simulink model "TargetTrackingRobotEnv"  (R2025a)
settings: Solver=VariableStepAuto  StartTime=0.0  StopTime=10.0  RelTol=1e-3
undefined symbols (not defined in the file): theta0, x0, y0
libraries: rllib x1
settings Model: Creator=ex  LastModifiedBy=ex

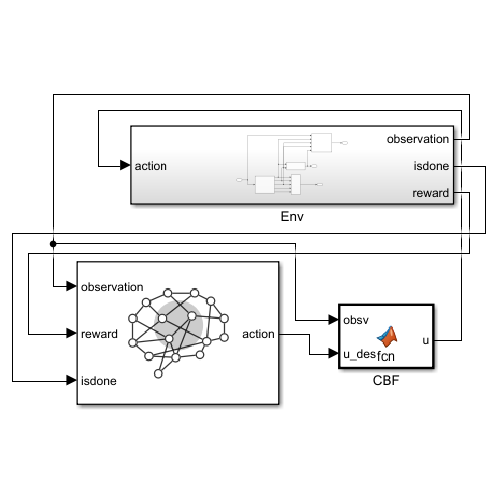
[thumbnail: Simulink's stored preview of the top-level diagram]
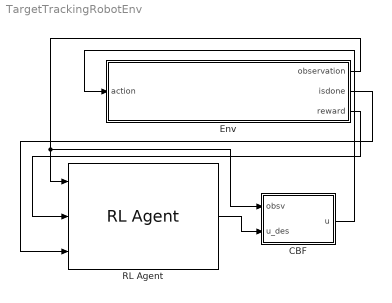
== system TargetTrackingRobotEnv ==
  CBF : MATLAB Function  TreatAsAtomicUnit=on
  Env : Subsystem
  RL Agent : rllib/RL Agent  Agent=agent  ExternalActionAsInput=off  ProvideLastAction=off  ProvideCumRwd=off  TreatAsDirectFeedthrough=on  UseStrictObservationDataTypes=off
  wires:
  Env/2(isdone) -> RL Agent/3
  Env/3(reward) -> RL Agent/2
  Env/1(observation) -> CBF/1(obsv), RL Agent/1
  RL Agent/1 -> CBF/2(u_des)
  CBF/1(u) -> Env/1(action)

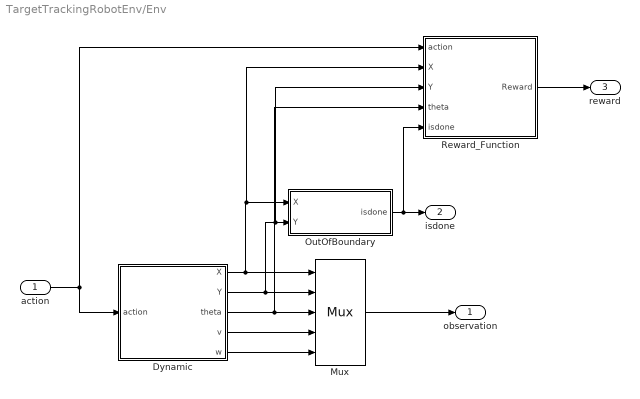
== system TargetTrackingRobotEnv/Env ==
  action : Inport
  Dynamic : Subsystem
  Mux : Mux  Inputs=5
  OutOfBoundary : Subsystem
  Reward_Function : Subsystem
  observation : Outport
  isdone : Outport  Port=2
  reward : Outport  Port=3
  wires:
  action/1 -> Reward_Function/1(action), Dynamic/1(action)
  Dynamic/1(X) -> Reward_Function/2(X), OutOfBoundary/1(X), Mux/1
  Dynamic/2(Y) -> Reward_Function/3(Y), OutOfBoundary/2(Y), Mux/2
  Dynamic/3(theta) -> Mux/3, Reward_Function/4(theta)
  Mux/1 -> observation/1
  OutOfBoundary/1(isdone) -> Reward_Function/5(isdone), isdone/1
  Reward_Function/1(Reward) -> reward/1
  Dynamic/4(v) -> Mux/4
  Dynamic/5(w) -> Mux/5

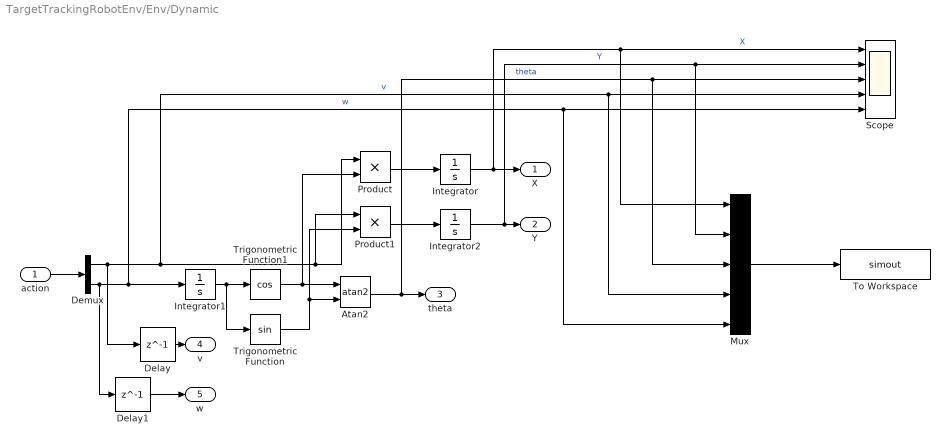
== system TargetTrackingRobotEnv/Env/Dynamic ==
  action : Inport
  Atan2 : Trigonometry  Operator=atan2
  Delay : Delay  DelayLength=1  InitialCondition=0
  Delay1 : Delay  DelayLength=1  InitialCondition=0
  Demux : Demux  Outputs=2
  Integrator : Integrator  InitialCondition=x0
  Integrator1 : Integrator  InitialCondition=theta0
  Integrator2 : Integrator  InitialCondition=y0
  Mux : Mux  Inputs=5
  Product : Product
  Product1 : Product
  Scope : Scope  NumInputPorts=5
      settings: ActiveDisplayYMinimum=-43.864327888983752  ActiveDisplayYMaximum=26.655261812730853
  To Workspace : ToWorkspace  VariableName=simout  SaveFormat=Structure With Time  SampleTime=-1
  Trigonometric Function : Trigonometry
  Trigonometric Function1 : Trigonometry  Operator=cos
  X : Outport
  Y : Outport  Port=2
  theta : Outport  Port=3
  v : Outport  Port=4
  w : Outport  Port=5
  wires:
  Trigonometric Function1/1 -> Product/2, Atan2/1
  Trigonometric Function/1 -> Product1/2, Atan2/2
  Demux/2 -> Mux/5, Scope/5, Integrator1/1, Delay1/1  "w"
  Demux/1 -> Delay/1, Mux/4, Scope/4, Product/1, Product1/1  "v"
  action/1 -> Demux/1
  Integrator1/1 -> Trigonometric Function/1, Trigonometric Function1/1
  Product1/1 -> Integrator2/1
  Integrator2/1 -> Mux/2, Scope/2, Y/1  "Y"
  Product/1 -> Integrator/1
  Integrator/1 -> Mux/1, Scope/1, X/1  "X"
  Atan2/1 -> Mux/3, Scope/3, theta/1  "theta"
  Delay/1 -> v/1
  Delay1/1 -> w/1
  Mux/1 -> To Workspace/1

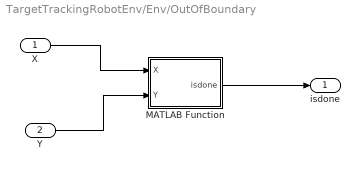
== system TargetTrackingRobotEnv/Env/OutOfBoundary ==
  X : Inport
  Y : Inport  Port=2
  MATLAB Function : MATLAB Function  TreatAsAtomicUnit=on
  isdone : Outport
  wires:
  X/1 -> MATLAB Function/1(X)
  Y/1 -> MATLAB Function/2(Y)
  MATLAB Function/1(isdone) -> isdone/1

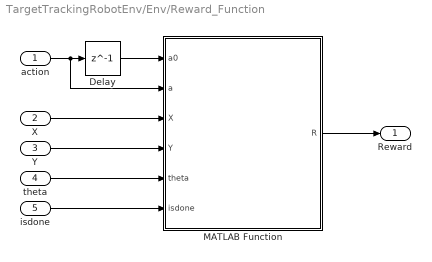
== system TargetTrackingRobotEnv/Env/Reward_Function ==
  action : Inport
  X : Inport  Port=2
  Y : Inport  Port=3
  theta : Inport  Port=4
  isdone : Inport  Port=5
  Delay : Delay  DelayLength=1  InitialCondition=0
  MATLAB Function : MATLAB Function  TreatAsAtomicUnit=on
  Reward : Outport
  wires:
  MATLAB Function/1(R) -> Reward/1
  action/1 -> MATLAB Function/2(a), Delay/1
  X/1 -> MATLAB Function/3(X)
  Y/1 -> MATLAB Function/4(Y)
  theta/1 -> MATLAB Function/5(theta)
  isdone/1 -> MATLAB Function/6(isdone)
  Delay/1 -> MATLAB Function/1(a0)

== matlab function TargetTrackingRobotEnv/Env/OutOfBoundary/MATLAB Function ==
  data: X input; isdone output; Y input
function isdone = fcn(X, Y)

boundary = 20;
isdone = false;
if abs(X) > boundary || abs(Y) > boundary
    isdone = true;
end

== matlab function TargetTrackingRobotEnv/Env/Reward_Function/MATLAB Function ==
  data: a0 input; a input; R output; X input; Y input; theta input; isdone input
function R = fcn(a0, a, X, Y, theta, isdone)

tarX = 0;
tarY = 0;
tarTheta = 0;

%Penalty of out of boundary
boundaryPenalty = 0;
if isdone 
    boundaryPenalty = -100;
end

% Reward for reaching near target position and orientation
distanceToTarget = 3*(X - tarX)^2 + 3*(Y - tarY)^2 ;
posR = 10 / (1 + 1 * distanceToTarget);
posP = -0.01 * distanceToTarget;
tarAngleR = 0;
if distanceToTarget < 0.5 && abs(tarTheta - theta) < 0.5
    tarAngleR = 5;
end

deltaV = (a0(2) - a(2))^2; 
% penalty for largest movement change
slowActionP = - 0.01 * deltaV;

% Penalize sharp turning
deltaW =(a0(2) - a(2))^2; 
sharpTuringP = -0.01*deltaW;

R = posR  + tarAngleR  + posP + boundaryPenalty + slowActionP  + sharpTuringP;

== matlab function TargetTrackingRobotEnv/CBF ==
  data: obsv input; u_des input; u output
function u = fcn(obsv, u_des)

x = obsv(1); 
y = obsv(2); 
theta = obsv(3); 

v_des = u_des(1);   
w_des = u_des(2);

% Obstacle parameters
xo = -4; 
yo = 0; 
ro  = 1.5;
safe_margin = 0.5;
r = ro + safe_margin;

% Barrier function and derivative term
h = (x - xo)^2 + (y - yo)^2 - r^2;
a = 2*((x - xo)*cos(theta) + (y - yo)*sin(theta));
gamma = 10;  

% Compute Psi
v_Psi = a*v_des + gamma*h;
w_Psi = a*w_des + gamma*h;

if (v_Psi < 0) 
    v =   gamma/a*h;
else
    v = v_des;
end

if (w_Psi < 0)
    w =  gamma/a*h;
else
    w = w_des;
end


u = zeros(2,1,'like',u_des); 
u(1) = v;
u(2) = w;

end
